simulink model "zhaojiajun0926"  (Simulink 8.5)
settings: Solver=ode113  StartTime=0.0  StopTime=1  MaxStep=0.0001  RelTol=1e-3
libraries: powerlib x6, powerlib_extras x3
settings Model: Creator=Administrator  LastModifiedBy=佳君
settings DebuggingCC: SolverPrmCheckMsg=warning  FcnCallInpInsideContextMsg=UseLocalSettings  StrictBusMsg=Warning

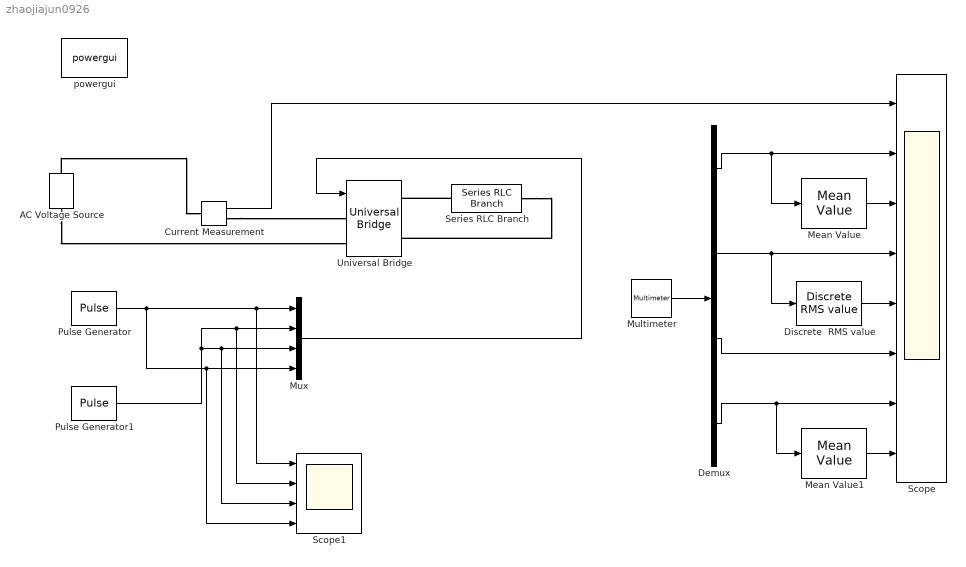
== system zhaojiajun0926 ==
  AC Voltage Source : powerlib/Electrical Sources/AC Voltage Source  Amplitude=220  Phase=0  Frequency=50  SampleTime=0  Measurements=Voltage
  Current Measurement : powerlib/Measurements/Current Measurement  PhasorSimulation=off  OutputType=Complex  PSBequivalent=0
  Demux : Demux
  Discrete  RMS value : powerlib_extras/Discrete Measurements/Discrete  RMS value  Freq=60  Mag_Init=0  Ts=50e-6
  Mean Value : powerlib_extras/Measurements/Mean Value  Period=1/60
  Mean Value1 : powerlib_extras/Measurements/Mean Value  Period=1/60
  Multimeter : powerlib/Measurements/Multimeter  PhasorSimulation=off  OutputType=Complex  sel=[1 10 2 9]  L=13  Gain=[1 1 1 1]  yselected={'Ub: Series RLC Branch','Isw1: Universal Bridge','Usw1: Universal Bridge','Ib: Series RLC Branch'};  PSBOutputType=1  PSBequivalent=0  AxesSetting=[0,0.1,-100,100]  Display=0  SavedBlockNames=-11
  Mux : Mux
  Pulse Generator : DiscretePulseGenerator  PulseType=Time based  Period=0.02  PulseWidth=10  PhaseDelay=0.00167
  Pulse Generator1 : DiscretePulseGenerator  PulseType=Time based  Period=0.02  PulseWidth=10  PhaseDelay=0.00167*2
  Scope : Scope  NumInputPorts=8
      settings: TimeRange=1  YMin=-5~-500~0~0~0~-500~-5~0  YMax=5~500~200~4~2~500~5~2
  Scope1 : Scope  NumInputPorts=4
      settings: TimeRange=1  YMin=-5~-5~-5~-5  YMax=5~5~5~5
  Series RLC Branch : powerlib/Elements/Series RLC Branch  LConnTagsString=__new0  RConnTagsString=__new0  BranchType=R  Resistance=100  Inductance=1e-3  SetiL0=off  InitialCurrent=0  Capacitance=1e-6  Setx0=off  InitialVoltage=0  Measurements=Branch voltage and current
  Universal Bridge : powerlib/Power Electronics/Universal Bridge  Arms=2  SnubberResistance=1e5  SnubberCapacitance=inf  Device=Thyristors  Ron=1e-3  Lon=0  ForwardVoltages="[  0  0  ]"  ForwardVoltage=0  GTOparameters=[ 10e-6 , 20e-6 ]  IGBTparameters=[ 1e-6 , 2e-6 ]  Measurements=All voltages and currents  Measurements_2=None  converterType=Rectifier
  powergui : powerlib/powergui  Priority=1  SimulationMode=Continuous  SolverType=Tustin/Backward Euler (TBE)  SampleTime=50e-6  frequency=60  SPID=off  DisableSnubberDevices=off  DisableRonSwitches=off  DisableVfSwitches=off  SwTol=0  DisplayEquations=off  Interpol=off  methode=off  Ts=0  FunctionMessages=off  echomessages=off  HookPort=off  EnableUseOfTLC=off  x0status=blocks  frequencyindice=50  Pbase=100e6  ErrMax=1e-4  Iterations=50  UnitsV=kV  UnitsW=MW  buscounter=0  RestoreLinks=warning  ResistiveCurrentMeasurement=off  Frange=[0:2:500]  Ylog=off  Xlog=on  ShowGrid=off  save=off  variable=ZData  structure=0  ZoomFFT=on  StartTime=0.0  cycles=1  DisplayStyle=1  fundamental=60  FreqAxis=off  MaxFrequency=1000  frequencyindicesteady=1  RmsSteady=1  display=off
  wires:
  Pulse Generator/1 -> Mux/1, Scope1/1, Mux/4, Scope1/4
  Pulse Generator1/1 -> Mux/2, Scope1/2, Mux/3, Scope1/3
  Mux/1 -> Universal Bridge/1
  Current Measurement/1 -> Scope/1
  Mean Value1/1 -> Scope/8
  Mean Value/1 -> Scope/3
  Demux/4 -> Mean Value1/1, Scope/7
  Demux/1 -> Mean Value/1, Scope/2
  Demux/3 -> Scope/6
  Discrete  RMS value/1 -> Scope/5
  Demux/2 -> Discrete  RMS value/1, Scope/4
  Multimeter/1 -> Demux/1
  connections:
  AC Voltage Source/RConn1 -- Current Measurement/LConn1
  AC Voltage Source/LConn1 -- Universal Bridge/LConn2
  Current Measurement/RConn1 -- Universal Bridge/LConn1
  Series RLC Branch/LConn1 -- Universal Bridge/RConn1
  Series RLC Branch/RConn1 -- Universal Bridge/RConn2
